simulink subsystem "ElectricalCoolingSystemSSC"  (R2022b)
settings: Solver=VariableStepAuto  StartTime=0.0  StopTime=10.0  RelTol=1e-3
undefined symbols (not defined in the file): BattTempInit, pipe, pump, radiator, T_env, T_set, tank, valve
libraries: fl_lib x101, nesl_utility_internal x25, SimscapeFluids_lib x7, slpidlib x1, simulink_extras x1
(part 2 of 3)

== system ElectricalCoolingSystemSSC/Air Stream ==
  V : Inport
  Air density [kg/m^3] : Constant  Value=1.225
  Air velocity [m/s] : Bias  Bias=5  SaturateOnIntegerOverflow=off
  Product : Product  Inputs=3
  Radiator area [m^2] : Constant  Value=radiator.area_air
  Simulink-PS Converter1 : nesl_utility_internal/Simulink-PS Converter  PhysicalDomain=network_engine_domain  SubClassName=ps_input  LeftPortType=input  RightPortType=output  PseudoPeriodic=off  Frequencies=[]  NoiseDistribution=none  NoiseParameters=[]  Unit=kg/s  AffineConversion=off  FilteringAndDerivatives=filter  SimscapeFilterOrder=1  InputFilterTimeConstant=0.01  UdotUserProvided=0
  mdot : PMIOPort  Side=Right
  wires:
  Air velocity [m/s]/1 -> Product/1
  Air density [kg/m^3]/1 -> Product/3
  Radiator area [m^2]/1 -> Product/2
  Product/1 -> Simulink-PS Converter1/1
  V/1 -> Air velocity [m/s]/1
  connections:
  mdot/RConn1 -- Simulink-PS Converter1/RConn1

== system ElectricalCoolingSystemSSC/Cold Plate ==
  One-Pass : Subsystem  VariantControl=1
  Inlet : PMIOPort  Side=Left
  Outlet : PMIOPort  Port=2  Side=Left
  Pack1 : PMIOPort  Port=3  Side=Right
  Pack2 : PMIOPort  Port=4  Side=Right
  Pack3 : PMIOPort  Port=5  Side=Right
  Pack4 : PMIOPort  Port=6  Side=Right

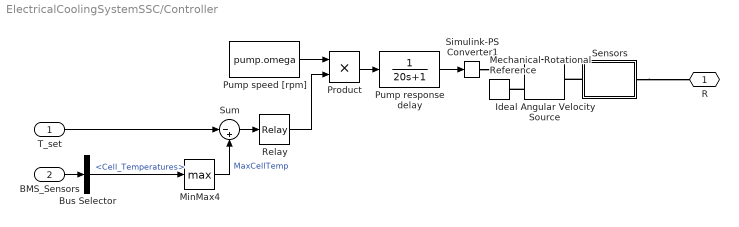
== system ElectricalCoolingSystemSSC/Controller ==
  T_set : Inport
  BMS_Sensors : Inport  Port=2
  Bus Selector : BusSelector  OutputSignals=Cell_Temperatures
  Ideal Angular Velocity Source : fl_lib/Mechanical/Mechanical Sources/Ideal Angular Velocity Source
  Mechanical Rotational Reference : fl_lib/Mechanical/Rotational Elements/Mechanical Rotational Reference
  MinMax4 : MinMax  Function=max
  Product : Product
  Pump response delay : TransferFcn  Denominator=[20 1]
  Pump speed [rpm] : Constant  Value=pump.omega
  Relay : Relay  OnSwitchValue=+1  OffSwitchValue=0.1
  Sensors : Subsystem
  Simulink-PS Converter1 : nesl_utility_internal/Simulink-PS Converter  PhysicalDomain=network_engine_domain  SubClassName=ps_input  LeftPortType=input  RightPortType=output  PseudoPeriodic=off  Frequencies=[]  NoiseDistribution=none  NoiseParameters=[]  Unit=rpm  AffineConversion=off  FilteringAndDerivatives=provide  SimscapeFilterOrder=1  InputFilterTimeConstant=0.001  UdotUserProvided=0
  Sum : Sum  Inputs=|-+
  R : PMIOPort  Side=Right
  wires:
  Pump response delay/1 -> Simulink-PS Converter1/1
  Product/1 -> Pump response delay/1
  Relay/1 -> Product/2
  Sum/1 -> Relay/1
  Pump speed [rpm]/1 -> Product/1
  T_set/1 -> Sum/1
  Bus Selector/1 -> MinMax4/1  "<Cell_Temperatures>"
  BMS_Sensors/1 -> Bus Selector/1
  MinMax4/1 -> Sum/2  "MaxCellTemp"
  connections:
  Sensors/LConn1 -- Ideal Angular Velocity Source/LConn1
  Simulink-PS Converter1/RConn1 -- Ideal Angular Velocity Source/RConn1
  Ideal Angular Velocity Source/RConn2 -- Mechanical Rotational Reference/LConn1
  Sensors/RConn1 -- R/RConn1

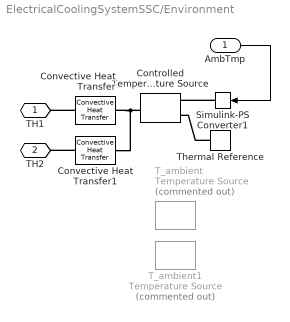
== system ElectricalCoolingSystemSSC/Environment ==
  AmbTmp : Inport
  Controlled Temperature Source : fl_lib/Thermal/Thermal Sources/Controlled Temperature Source
  Convective Heat Transfer : fl_lib/Thermal/Thermal Elements/Convective Heat Transfer  thermal_type=foundation.enum.constant_variable.constant  area=tank.area_wall/2 m^2  heat_tr_coeff=20 W/(m^2 * K)  min_heat_tr_coeff=1e-3 W/(K*m^2)  T_specify=off  T_priority=None  T=0 K  T_nominal_specify=off  T_nominal_unit=K  T_nominal_value=1  Q_specify=off  Q_priority=None  Q=0 W  Q_nominal_specify=off  Q_nominal_unit=W  Q_nominal_value=1
  Convective Heat Transfer1 : fl_lib/Thermal/Thermal Elements/Convective Heat Transfer  thermal_type=foundation.enum.constant_variable.constant  area=tank.area_wall/2 m^2  heat_tr_coeff=20 W/(m^2 * K)  min_heat_tr_coeff=1e-3 W/(K*m^2)  T_specify=off  T_priority=None  T=0 K  T_nominal_specify=off  T_nominal_unit=K  T_nominal_value=1  Q_specify=off  Q_priority=None  Q=0 W  Q_nominal_specify=off  Q_nominal_unit=W  Q_nominal_value=1
  Simulink-PS Converter1 : nesl_utility_internal/Simulink-PS Converter  PhysicalDomain=network_engine_domain  SubClassName=ps_input  LeftPortType=input  RightPortType=output  PseudoPeriodic=off  Frequencies=[]  NoiseDistribution=none  NoiseParameters=[]  Unit=1  AffineConversion=off  FilteringAndDerivatives=provide  SimscapeFilterOrder=1  InputFilterTimeConstant=0.001  UdotUserProvided=0
  T_ambient : fl_lib/Thermal/Thermal Sources/Temperature Source  Commented=on  temperature=T_env degC
  T_ambient1 : fl_lib/Thermal/Thermal Sources/Temperature Source  Commented=on  temperature=T_env degC
  Thermal Reference : fl_lib/Thermal/Thermal Elements/Thermal Reference
  TH1 : PMIOPort  Side=Left
  TH2 : PMIOPort  Port=2  Side=Left
  wires:
  AmbTmp/1 -> Simulink-PS Converter1/1
  connections:
  Convective Heat Transfer/LConn1 -- TH1/RConn1
  Convective Heat Transfer1/LConn1 -- TH2/RConn1
  Convective Heat Transfer/RConn1 -- Controlled Temperature Source/LConn1 -- Convective Heat Transfer1/RConn1
  Simulink-PS Converter1/RConn1 -- Controlled Temperature Source/RConn1
  Thermal Reference/LConn1 -- Controlled Temperature Source/RConn2

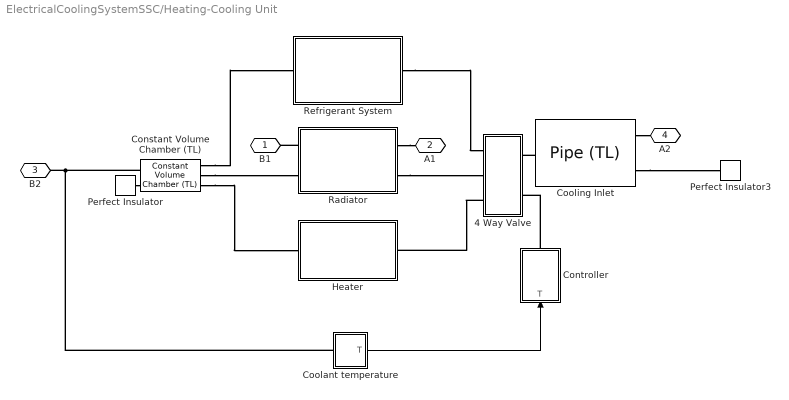
== system ElectricalCoolingSystemSSC/Heating-Cooling Unit ==
  4 Way Valve : Subsystem
  Constant Volume Chamber (TL) : fl_lib/Thermal Liquid/Elements/Constant Volume Chamber (TL)  volume=5 cm^3  num_ports=foundation.enum.num_ports.four  area_A=pipe.area m^2  area_B=pipe.area*10 m^2  area_C=pipe.area m^2  area_D=pipe.area m^2  p_I_specify=off  p_I_priority=High  p_I=0.101325 MPa  p_I_nominal_specify=off  p_I_nominal_unit=MPa  p_I_nominal_value=1  T_I_specify=on  T_I_priority=High  T_I=BattTempInit degC  T_I_nominal_specify=off  T_I_nominal_unit=K  T_I_nominal_value=1  u_chamber_specify=off  u_chamber_priority=None  u_chamber=83.90600000000001 kJ/kg  u_chamber_nominal_specify=off  u_chamber_nominal_unit=kJ/kg  u_chamber_nominal_value=1  rho_specify=off  rho_priority=None  rho=998.21 kg/m^3  rho_nominal_specify=off  rho_nominal_unit=kg/m^3  rho_nominal_value=1
      settings: InternalSimscapePortConfiguration="{\"Bottom\":[],\"Left\":[{\"id\":\"A\",\"label\":\"A\",\"type\":\"foundation.thermal_liquid.thermal_liquid\"},{\"id\":\"H\",\"label\":\"H\",\"type\":\"foundation.thermal.thermal\"}],\"Right\":[{\"id\":\"B\",\"label\":\"B\",\"type\":\"foundation.thermal_liquid.thermal_liquid\"},{\"id\":\"C\",\"label\":\"C\",\"type\":\"foundation.thermal_liquid.thermal_liquid\"},{\"id\":\"D\",\"label\":\"D\",\"type\":\"foundation.thermal_liquid.thermal_liquid\"}],\"Top\":[]}"
  Controller : Subsystem
  Coolant temperature : Subsystem
  Cooling Inlet : fl_lib/Thermal Liquid/Elements/Pipe (TL)  length=0.75 m  area=pipe.area cm^2  Dh=pipe.Dh cm  length_add=0 m  roughness=15e-6 m  Re_lam=2000  Re_tur=4000  shape_factor=64  Nu_lam=3.66  dynamic_compressibility=simscape.enum.onoff.on  inertia=simscape.enum.onoff.off  p0=0.101325 MPa  T0=BattTempInit degC  mdot0=0 kg/s
  Heater : Subsystem
  Perfect Insulator : fl_lib/Thermal/Thermal Elements/Perfect Insulator  T_specify=off  T_priority=None  T=0 K  T_nominal_specify=off  T_nominal_unit=K  T_nominal_value=1
  Perfect Insulator3 : fl_lib/Thermal/Thermal Elements/Perfect Insulator  T_specify=off  T_priority=None  T=0 K  T_nominal_specify=off  T_nominal_unit=K  T_nominal_value=1
  Radiator : Subsystem
  Refrigerant System : Subsystem
  B1 : PMIOPort  Side=Right
  A1 : PMIOPort  Port=2  Side=Left
  B2 : PMIOPort  Port=3  Side=Left
  A2 : PMIOPort  Port=4  Side=Right
  wires:
  Coolant temperature/1(T) -> Controller/1(T)
  connections:
  Constant Volume Chamber (TL)/RConn2 -- Radiator/LConn2
  4 Way Valve/LConn3 -- Heater/RConn1
  B2/RConn1 -- Coolant temperature/LConn1 -- Constant Volume Chamber (TL)/LConn1
  Constant Volume Chamber (TL)/RConn3 -- Heater/LConn1
  Radiator/LConn1 -- B1/RConn1
  Refrigerant System/RConn1 -- 4 Way Valve/LConn1
  Radiator/RConn1 -- A1/RConn1
  Cooling Inlet/LConn1 -- A2/RConn1
  Cooling Inlet/RConn1 -- 4 Way Valve/RConn1
  Radiator/RConn2 -- 4 Way Valve/LConn2
  Controller/RConn1 -- 4 Way Valve/RConn2
  Constant Volume Chamber (TL)/RConn1 -- Refrigerant System/LConn1
  Cooling Inlet/LConn2 -- Perfect Insulator3/LConn1
  Perfect Insulator/LConn1 -- Constant Volume Chamber (TL)/LConn2

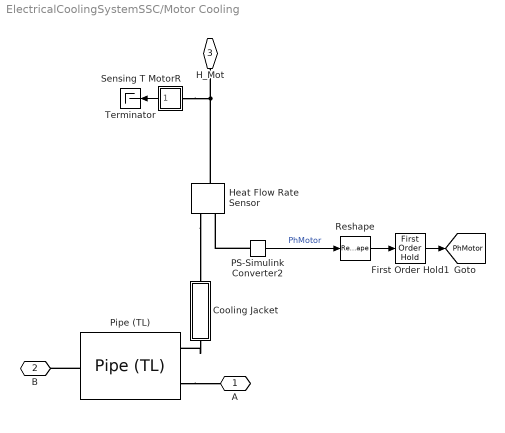
== system ElectricalCoolingSystemSSC/Motor Cooling ==
  Cooling Jacket : Subsystem
  First Order Hold1 : FirstOrderHold  ErrorTolerance=inf  AllowContinuousInput=on
  Heat Flow Rate Sensor : fl_lib/Thermal/Thermal Sensors/Heat Flow Rate Sensor
  PS-Simulink Converter2 : nesl_utility_internal/PS-Simulink Converter  PhysicalDomain=network_engine_domain  SubClassName=ps_output  LeftPortType=input  RightPortType=output  PseudoPeriodic=off  Frequencies=[]  VectorFormat=inherit  Unit=inherit  AffineConversion=off
  Pipe (TL) : fl_lib/Thermal Liquid/Elements/Pipe (TL)  length=pipe.length cm  area=pipe.area cm^2  Dh=pipe.Dh cm  length_add=0 m  roughness=15e-6 m  Re_lam=2000  Re_tur=4000  shape_factor=64  Nu_lam=3.66  dynamic_compressibility=simscape.enum.onoff.on  inertia=simscape.enum.onoff.off  p0=0.101325 MPa  T0=BattTempInit degC  mdot0=0 kg/s
  Reshape : Reshape
  Sensing T MotorR : Subsystem
  Terminator : Terminator
  A : PMIOPort  Side=Left
  B : PMIOPort  Port=2  Side=Right
  H_Mot : PMIOPort  Port=3  Side=Right
  tag scope: PhMotor=global
  wires:
  Sensing T MotorR/1(T) -> Terminator/1
  PS-Simulink Converter2/1 -> Reshape/1  "PhMotor"
  Reshape/1 -> First Order Hold1/1
  First Order Hold1/1 -> [PhMotor]
  connections:
  Pipe (TL)/RConn1 -- B/RConn1
  Pipe (TL)/LConn1 -- A/RConn1
  Sensing T MotorR/LConn1 -- H_Mot/RConn1 -- Heat Flow Rate Sensor/LConn1
  Cooling Jacket/LConn1 -- Pipe (TL)/LConn2
  PS-Simulink Converter2/LConn1 -- Heat Flow Rate Sensor/RConn1
  Heat Flow Rate Sensor/RConn2 -- Cooling Jacket/RConn1

== system ElectricalCoolingSystemSSC/Power Sensor ==
  First Order Hold1 : FirstOrderHold  ErrorTolerance=inf  AllowContinuousInput=on
  Heat Flow Rate Sensor : fl_lib/Thermal/Thermal Sensors/Heat Flow Rate Sensor
  PS-Simulink Converter2 : nesl_utility_internal/PS-Simulink Converter  PhysicalDomain=network_engine_domain  SubClassName=ps_output  LeftPortType=input  RightPortType=output  PseudoPeriodic=off  Frequencies=[]  VectorFormat=inherit  Unit=inherit  AffineConversion=off
  Reshape : Reshape
  A : PMIOPort  Side=Left
  B : PMIOPort  Port=2  Side=Right
  tag scope: Ph1=global
  wires:
  PS-Simulink Converter2/1 -> Reshape/1  "Ph1"
  Reshape/1 -> First Order Hold1/1
  First Order Hold1/1 -> [Ph1]
  connections:
  PS-Simulink Converter2/LConn1 -- Heat Flow Rate Sensor/RConn1
  Heat Flow Rate Sensor/LConn1 -- A/RConn1
  Heat Flow Rate Sensor/RConn2 -- B/RConn1

== system ElectricalCoolingSystemSSC/Power Sensor1 ==
  First Order Hold1 : FirstOrderHold  ErrorTolerance=inf  AllowContinuousInput=on
  Mass & Energy Flow Rate Sensor (TL) : fl_lib/Thermal Liquid/Sensors/Mass & Energy Flow Rate Sensor (TL)
      settings: InternalSimscapePortConfiguration="{\"Bottom\":[],\"Left\":[{\"id\":\"A\",\"label\":\"A\",\"type\":\"foundation.thermal_liquid.thermal_liquid\"}],\"Right\":[{\"id\":\"B\",\"label\":\"B\",\"type\":\"foundation.thermal_liquid.thermal_liquid\"},{\"id\":\"M\",\"label\":\"M\",\"type\":\"output\"},{\"id\":\"PHI\",\"label\":\"Phi\",\"type\":\"output\"}],\"Top\":[]}"
  PS-Simulink Converter2 : nesl_utility_internal/PS-Simulink Converter  PhysicalDomain=network_engine_domain  SubClassName=ps_output  LeftPortType=input  RightPortType=output  PseudoPeriodic=off  Frequencies=[]  VectorFormat=inherit  Unit=inherit  AffineConversion=off
  Reshape : Reshape
  B : PMIOPort  Side=Left
  A : PMIOPort  Port=2  Side=Right
  tag scope: PcpOutlet=global
  wires:
  PS-Simulink Converter2/1 -> Reshape/1  "PcpOutlet"
  Reshape/1 -> First Order Hold1/1
  First Order Hold1/1 -> [PcpOutlet]
  connections:
  Mass & Energy Flow Rate Sensor (TL)/RConn1 -- B/RConn1
  Mass & Energy Flow Rate Sensor (TL)/RConn3 -- PS-Simulink Converter2/LConn1
  Mass & Energy Flow Rate Sensor (TL)/LConn1 -- A/RConn1

== system ElectricalCoolingSystemSSC/Power Sensor2 ==
  First Order Hold1 : FirstOrderHold  ErrorTolerance=inf  AllowContinuousInput=on
  Mass & Energy Flow Rate Sensor (TL) : fl_lib/Thermal Liquid/Sensors/Mass & Energy Flow Rate Sensor (TL)
      settings: InternalSimscapePortConfiguration="{\"Bottom\":[],\"Left\":[{\"id\":\"A\",\"label\":\"A\",\"type\":\"foundation.thermal_liquid.thermal_liquid\"}],\"Right\":[{\"id\":\"B\",\"label\":\"B\",\"type\":\"foundation.thermal_liquid.thermal_liquid\"},{\"id\":\"M\",\"label\":\"M\",\"type\":\"output\"},{\"id\":\"PHI\",\"label\":\"Phi\",\"type\":\"output\"}],\"Top\":[]}"
  PS-Simulink Converter2 : nesl_utility_internal/PS-Simulink Converter  PhysicalDomain=network_engine_domain  SubClassName=ps_output  LeftPortType=input  RightPortType=output  PseudoPeriodic=off  Frequencies=[]  VectorFormat=inherit  Unit=inherit  AffineConversion=off
  Reshape : Reshape
  B : PMIOPort  Side=Left
  A : PMIOPort  Port=2  Side=Right
  tag scope: PhcuOut=global
  wires:
  PS-Simulink Converter2/1 -> Reshape/1  "PhcuOut"
  Reshape/1 -> First Order Hold1/1
  First Order Hold1/1 -> [PhcuOut]
  connections:
  Mass & Energy Flow Rate Sensor (TL)/LConn1 -- A/RConn1
  Mass & Energy Flow Rate Sensor (TL)/RConn3 -- PS-Simulink Converter2/LConn1
  Mass & Energy Flow Rate Sensor (TL)/RConn1 -- B/RConn1

== system ElectricalCoolingSystemSSC/Power Sensor3 ==
  First Order Hold1 : FirstOrderHold  ErrorTolerance=inf  AllowContinuousInput=on
  Mass & Energy Flow Rate Sensor (TL) : fl_lib/Thermal Liquid/Sensors/Mass & Energy Flow Rate Sensor (TL)
      settings: InternalSimscapePortConfiguration="{\"Bottom\":[],\"Left\":[{\"id\":\"A\",\"label\":\"A\",\"type\":\"foundation.thermal_liquid.thermal_liquid\"}],\"Right\":[{\"id\":\"B\",\"label\":\"B\",\"type\":\"foundation.thermal_liquid.thermal_liquid\"},{\"id\":\"M\",\"label\":\"M\",\"type\":\"output\"},{\"id\":\"PHI\",\"label\":\"Phi\",\"type\":\"output\"}],\"Top\":[]}"
  PS-Simulink Converter2 : nesl_utility_internal/PS-Simulink Converter  PhysicalDomain=network_engine_domain  SubClassName=ps_output  LeftPortType=input  RightPortType=output  PseudoPeriodic=off  Frequencies=[]  VectorFormat=inherit  Unit=inherit  AffineConversion=off
  Reshape : Reshape
  B : PMIOPort  Side=Left
  A : PMIOPort  Port=2  Side=Right
  tag scope: PhcuIn=global
  wires:
  PS-Simulink Converter2/1 -> Reshape/1  "PhcuIn"
  Reshape/1 -> First Order Hold1/1
  First Order Hold1/1 -> [PhcuIn]
  connections:
  Mass & Energy Flow Rate Sensor (TL)/LConn1 -- A/RConn1
  Mass & Energy Flow Rate Sensor (TL)/RConn3 -- PS-Simulink Converter2/LConn1
  Mass & Energy Flow Rate Sensor (TL)/RConn1 -- B/RConn1

== system ElectricalCoolingSystemSSC/Power Sensor4 ==
  First Order Hold1 : FirstOrderHold  ErrorTolerance=inf  AllowContinuousInput=on
  Mass & Energy Flow Rate Sensor (TL) : fl_lib/Thermal Liquid/Sensors/Mass & Energy Flow Rate Sensor (TL)
      settings: InternalSimscapePortConfiguration="{\"Bottom\":[],\"Left\":[{\"id\":\"A\",\"label\":\"A\",\"type\":\"foundation.thermal_liquid.thermal_liquid\"}],\"Right\":[{\"id\":\"B\",\"label\":\"B\",\"type\":\"foundation.thermal_liquid.thermal_liquid\"},{\"id\":\"M\",\"label\":\"M\",\"type\":\"output\"},{\"id\":\"PHI\",\"label\":\"Phi\",\"type\":\"output\"}],\"Top\":[]}"
  PS-Simulink Converter2 : nesl_utility_internal/PS-Simulink Converter  PhysicalDomain=network_engine_domain  SubClassName=ps_output  LeftPortType=input  RightPortType=output  PseudoPeriodic=off  Frequencies=[]  VectorFormat=inherit  Unit=inherit  AffineConversion=off
  Reshape : Reshape
  B : PMIOPort  Side=Left
  A : PMIOPort  Port=2  Side=Right
  tag scope: PMotOut=global
  wires:
  PS-Simulink Converter2/1 -> Reshape/1  "PMotOut"
  Reshape/1 -> First Order Hold1/1
  First Order Hold1/1 -> [PMotOut]
  connections:
  Mass & Energy Flow Rate Sensor (TL)/LConn1 -- A/RConn1
  Mass & Energy Flow Rate Sensor (TL)/RConn3 -- PS-Simulink Converter2/LConn1
  Mass & Energy Flow Rate Sensor (TL)/RConn1 -- B/RConn1

== system ElectricalCoolingSystemSSC/Power Sensor6 ==
  First Order Hold1 : FirstOrderHold  ErrorTolerance=inf  AllowContinuousInput=on
  Heat Flow Rate Sensor : fl_lib/Thermal/Thermal Sensors/Heat Flow Rate Sensor
  PS-Simulink Converter2 : nesl_utility_internal/PS-Simulink Converter  PhysicalDomain=network_engine_domain  SubClassName=ps_output  LeftPortType=input  RightPortType=output  PseudoPeriodic=off  Frequencies=[]  VectorFormat=inherit  Unit=inherit  AffineConversion=off
  Reshape : Reshape
  A : PMIOPort  Side=Left
  B : PMIOPort  Port=2  Side=Right
  tag scope: Ph2=global
  wires:
  PS-Simulink Converter2/1 -> Reshape/1
  Reshape/1 -> First Order Hold1/1
  First Order Hold1/1 -> [Ph2]
  connections:
  Heat Flow Rate Sensor/RConn2 -- B/RConn1
  Heat Flow Rate Sensor/LConn1 -- A/RConn1
  PS-Simulink Converter2/LConn1 -- Heat Flow Rate Sensor/RConn1

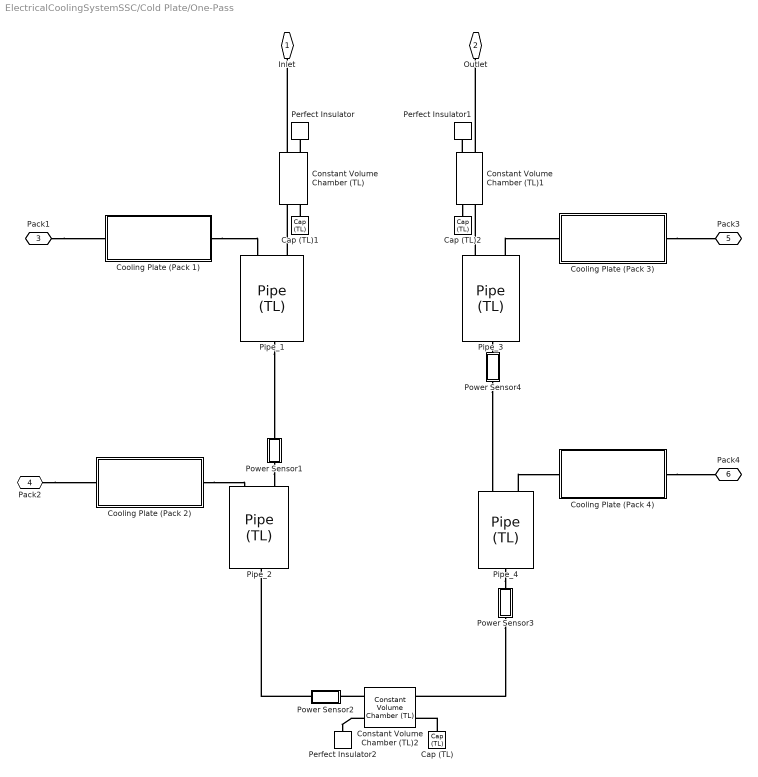
== system ElectricalCoolingSystemSSC/Cold Plate/One-Pass ==
  Cap (TL) : fl_lib/Thermal Liquid/Elements/Cap (TL)  p_specify=off  p_priority=None  p=0.101325 MPa  p_nominal_specify=off  p_nominal_unit=MPa  p_nominal_value=1  T_specify=off  T_priority=None  T=293.15 K  T_nominal_specify=off  T_nominal_unit=K  T_nominal_value=1
      settings: InternalSimscapePortConfiguration="{\"Bottom\":[],\"Left\":[{\"id\":\"A\",\"label\":\"\",\"type\":\"foundation.thermal_liquid.thermal_liquid\"}],\"Right\":[],\"Top\":[]}"
  Cap (TL)1 : fl_lib/Thermal Liquid/Elements/Cap (TL)  p_specify=off  p_priority=None  p=0.101325 MPa  p_nominal_specify=off  p_nominal_unit=MPa  p_nominal_value=1  T_specify=off  T_priority=None  T=293.15 K  T_nominal_specify=off  T_nominal_unit=K  T_nominal_value=1
      settings: InternalSimscapePortConfiguration="{\"Bottom\":[],\"Left\":[{\"id\":\"A\",\"label\":\"\",\"type\":\"foundation.thermal_liquid.thermal_liquid\"}],\"Right\":[],\"Top\":[]}"
  Cap (TL)2 : fl_lib/Thermal Liquid/Elements/Cap (TL)  p_specify=off  p_priority=None  p=0.101325 MPa  p_nominal_specify=off  p_nominal_unit=MPa  p_nominal_value=1  T_specify=off  T_priority=None  T=293.15 K  T_nominal_specify=off  T_nominal_unit=K  T_nominal_value=1
      settings: InternalSimscapePortConfiguration="{\"Bottom\":[],\"Left\":[{\"id\":\"A\",\"label\":\"\",\"type\":\"foundation.thermal_liquid.thermal_liquid\"}],\"Right\":[],\"Top\":[]}"
  Constant Volume Chamber (TL) : fl_lib/Thermal Liquid/Elements/Constant Volume Chamber (TL)  volume=0.001 m^3  num_ports=foundation.enum.num_ports.three  area_A=3 cm^2  area_B=3 cm^2  area_C=3 cm^2  area_D=0.01 m^2  p_I_specify=off  p_I_priority=High  p_I=0.101325 MPa  p_I_nominal_specify=off  p_I_nominal_unit=MPa  p_I_nominal_value=1  T_I_specify=on  T_I_priority=High  T_I=BattTempInit degC  T_I_nominal_specify=off  T_I_nominal_unit=K  T_I_nominal_value=1  u_chamber_specify=off  u_chamber_priority=None  u_chamber=83.90600000000001 kJ/kg  u_chamber_nominal_specify=off  u_chamber_nominal_unit=kJ/kg  u_chamber_nominal_value=1  rho_specify=off  rho_priority=None  rho=998.21 kg/m^3  rho_nominal_specify=off  rho_nominal_unit=kg/m^3  rho_nominal_value=1
      settings: InternalSimscapePortConfiguration="{\"Bottom\":[],\"Left\":[{\"id\":\"A\",\"label\":\"A\",\"type\":\"foundation.thermal_liquid.thermal_liquid\"},{\"id\":\"H\",\"label\":\"H\",\"type\":\"foundation.thermal.thermal\"}],\"Right\":[{\"id\":\"B\",\"label\":\"B\",\"type\":\"foundation.thermal_liquid.thermal_liquid\"},{\"id\":\"C\",\"label\":\"C\",\"type\":\"foundation.thermal_liquid.thermal_liquid\"}],\"Top\":[]}"
  Constant Volume Chamber (TL)1 : fl_lib/Thermal Liquid/Elements/Constant Volume Chamber (TL)  volume=0.001 m^3  num_ports=foundation.enum.num_ports.three  area_A=3 cm^2  area_B=3 cm^2  area_C=3 cm^2  area_D=0.01 m^2  p_I_specify=off  p_I_priority=High  p_I=0.101325 MPa  p_I_nominal_specify=off  p_I_nominal_unit=MPa  p_I_nominal_value=1  T_I_specify=on  T_I_priority=High  T_I=BattTempInit degC  T_I_nominal_specify=off  T_I_nominal_unit=K  T_I_nominal_value=1  u_chamber_specify=off  u_chamber_priority=None  u_chamber=83.90600000000001 kJ/kg  u_chamber_nominal_specify=off  u_chamber_nominal_unit=kJ/kg  u_chamber_nominal_value=1  rho_specify=off  rho_priority=None  rho=998.21 kg/m^3  rho_nominal_specify=off  rho_nominal_unit=kg/m^3  rho_nominal_value=1
      settings: InternalSimscapePortConfiguration="{\"Bottom\":[],\"Left\":[{\"id\":\"A\",\"label\":\"A\",\"type\":\"foundation.thermal_liquid.thermal_liquid\"},{\"id\":\"H\",\"label\":\"H\",\"type\":\"foundation.thermal.thermal\"}],\"Right\":[{\"id\":\"B\",\"label\":\"B\",\"type\":\"foundation.thermal_liquid.thermal_liquid\"},{\"id\":\"C\",\"label\":\"C\",\"type\":\"foundation.thermal_liquid.thermal_liquid\"}],\"Top\":[]}"
  Constant Volume Chamber (TL)2 : fl_lib/Thermal Liquid/Elements/Constant Volume Chamber (TL)  volume=0.001 m^3  num_ports=foundation.enum.num_ports.three  area_A=3 cm^2  area_B=3 cm^2  area_C=3 cm^2  area_D=0.01 m^2  p_I_specify=off  p_I_priority=High  p_I=0.101325 MPa  p_I_nominal_specify=off  p_I_nominal_unit=MPa  p_I_nominal_value=1  T_I_specify=on  T_I_priority=High  T_I=BattTempInit degC  T_I_nominal_specify=off  T_I_nominal_unit=K  T_I_nominal_value=1  u_chamber_specify=off  u_chamber_priority=None  u_chamber=83.90600000000001 kJ/kg  u_chamber_nominal_specify=off  u_chamber_nominal_unit=kJ/kg  u_chamber_nominal_value=1  rho_specify=off  rho_priority=None  rho=998.21 kg/m^3  rho_nominal_specify=off  rho_nominal_unit=kg/m^3  rho_nominal_value=1
      settings: InternalSimscapePortConfiguration="{\"Bottom\":[],\"Left\":[{\"id\":\"A\",\"label\":\"A\",\"type\":\"foundation.thermal_liquid.thermal_liquid\"},{\"id\":\"H\",\"label\":\"H\",\"type\":\"foundation.thermal.thermal\"}],\"Right\":[{\"id\":\"B\",\"label\":\"B\",\"type\":\"foundation.thermal_liquid.thermal_liquid\"},{\"id\":\"C\",\"label\":\"C\",\"type\":\"foundation.thermal_liquid.thermal_liquid\"}],\"Top\":[]}"
  Cooling Plate (Pack 1) : Subsystem
  Cooling Plate (Pack 2) : Subsystem
  Cooling Plate (Pack 3) : Subsystem
  Cooling Plate (Pack 4) : Subsystem
  Perfect Insulator : fl_lib/Thermal/Thermal Elements/Perfect Insulator  T_specify=off  T_priority=None  T=0 K  T_nominal_specify=off  T_nominal_unit=K  T_nominal_value=1
  Perfect Insulator1 : fl_lib/Thermal/Thermal Elements/Perfect Insulator  T_specify=off  T_priority=None  T=0 K  T_nominal_specify=off  T_nominal_unit=K  T_nominal_value=1
  Perfect Insulator2 : fl_lib/Thermal/Thermal Elements/Perfect Insulator  T_specify=off  T_priority=None  T=0 K  T_nominal_specify=off  T_nominal_unit=K  T_nominal_value=1
  Pipe_{1..4} (4 alike) : fl_lib/Thermal Liquid/Elements/Pipe (TL)  length=1.5 m  area=3*2 cm^2  Dh=0.92*sqrt(2) cm  length_add=0 m  roughness=15e-6 m  Re_lam=2000  Re_tur=4000  shape_factor=64  Nu_lam=3.66  dynamic_compressibility=simscape.enum.onoff.on  inertia=simscape.enum.onoff.off  p0=0.101325 MPa  T0=BattTempInit degC  mdot0=0 kg/s
  Power Sensor1 : Subsystem
  Power Sensor2 : Subsystem
  Power Sensor3 : Subsystem
  Power Sensor4 : Subsystem
  Inlet : PMIOPort  Side=Left
  Outlet : PMIOPort  Port=2  Side=Left
  Pack1 : PMIOPort  Port=3  Side=Right
  Pack2 : PMIOPort  Port=4  Side=Right
  Pack3 : PMIOPort  Port=5  Side=Right
  Pack4 : PMIOPort  Port=6  Side=Right
  connections:
  Constant Volume Chamber (TL)1/RConn2 -- Cap (TL)2/LConn1
  Cap (TL)1/LConn1 -- Constant Volume Chamber (TL)/RConn2
  Cap (TL)/LConn1 -- Constant Volume Chamber (TL)2/RConn2
  Pipe_3/RConn1 -- Power Sensor4/RConn1
  Constant Volume Chamber (TL)2/LConn1 -- Power Sensor2/RConn1
  Constant Volume Chamber (TL)/LConn1 -- Inlet/RConn1
  Constant Volume Chamber (TL)1/LConn2 -- Perfect Insulator1/LConn1
  Power Sensor3/LConn1 -- Constant Volume Chamber (TL)2/RConn1
  Constant Volume Chamber (TL)1/LConn1 -- Outlet/RConn1
  Pack1/RConn1 -- Cooling Plate (Pack 1)/RConn1
  Pack2/RConn1 -- Cooling Plate (Pack 2)/RConn1
  Pipe_1/RConn1 -- Power Sensor1/RConn1
  Pipe_3/LConn1 -- Constant Volume Chamber (TL)1/RConn1
  Pipe_3/LConn2 -- Cooling Plate (Pack 3)/LConn1
  Pipe_4/LConn2 -- Cooling Plate (Pack 4)/LConn1
  Cooling Plate (Pack 1)/LConn1 -- Pipe_1/LConn2
  Cooling Plate (Pack 2)/LConn1 -- Pipe_2/LConn2
  Cooling Plate (Pack 3)/RConn1 -- Pack3/RConn1
  Cooling Plate (Pack 4)/RConn1 -- Pack4/RConn1
  Power Sensor1/LConn1 -- Pipe_2/LConn1
  Power Sensor4/LConn1 -- Pipe_4/LConn1
  Power Sensor2/LConn1 -- Pipe_2/RConn1
  Pipe_4/RConn1 -- Power Sensor3/RConn1
  Constant Volume Chamber (TL)2/LConn2 -- Perfect Insulator2/LConn1
  Pipe_1/LConn1 -- Constant Volume Chamber (TL)/RConn1
  Constant Volume Chamber (TL)/LConn2 -- Perfect Insulator/LConn1

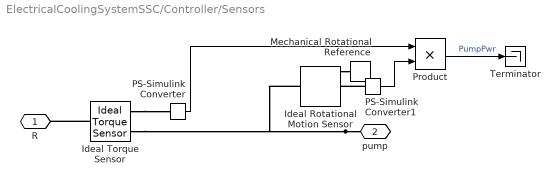
== system ElectricalCoolingSystemSSC/Controller/Sensors ==
  Ideal Rotational Motion Sensor : fl_lib/Mechanical/Mechanical Sensors/Ideal Rotational Motion Sensor  reference=foundation.enum.MeasurementReference.difference  acceleration_port=false  velocity_port=true  position_port=true  wrap_angle=simscape.enum.onoff.off  offset=0 rad
  Ideal Torque Sensor : fl_lib/Mechanical/Mechanical Sensors/Ideal Torque Sensor
  Mechanical Rotational Reference : fl_lib/Mechanical/Rotational Elements/Mechanical Rotational Reference
  PS-Simulink Converter : nesl_utility_internal/PS-Simulink Converter  PhysicalDomain=network_engine_domain  SubClassName=ps_output  LeftPortType=input  RightPortType=output  PseudoPeriodic=off  Frequencies=[]  VectorFormat=1-D array  Unit=N*m  AffineConversion=off
  PS-Simulink Converter1 : nesl_utility_internal/PS-Simulink Converter  PhysicalDomain=network_engine_domain  SubClassName=ps_output  LeftPortType=input  RightPortType=output  PseudoPeriodic=off  Frequencies=[]  VectorFormat=1-D array  Unit=rad/s  AffineConversion=off
  Product : Product
  Terminator : Terminator
  R : PMIOPort  Side=Left
  pump : PMIOPort  Port=2  Side=Right
  wires:
  PS-Simulink Converter/1 -> Product/1
  PS-Simulink Converter1/1 -> Product/2
  Product/1 -> Terminator/1  "PumpPwr"
  connections:
  Ideal Rotational Motion Sensor/RConn1 -- Mechanical Rotational Reference/LConn1
  Ideal Torque Sensor/LConn1 -- R/RConn1
  Ideal Torque Sensor/RConn2 -- PS-Simulink Converter/LConn1
  PS-Simulink Converter1/LConn1 -- Ideal Rotational Motion Sensor/RConn2
  pump/RConn1 -- Ideal Rotational Motion Sensor/LConn1 -- Ideal Torque Sensor/RConn1

== system ElectricalCoolingSystemSSC/Heating-Cooling Unit/4 Way Valve ==
  Variable Area Orifice (TL) : SimscapeFluids_lib/Thermal Liquid/Valves & Orifices/Orifice (TL)  orifice_type=foundation.enum.constant_variable.variable  constant_orifice_spec=fluids.thermal_liquid.valves.enum.ConstantOrificeSpec.Area  variable_orifice_spec=2  orifice_area_constant=1e-3 m^2  p_diff_TLU_constant=[-4, -3, -2, -1, -.5, 0, .5, 1, 2, 3, 4] MPa  vol_flow_TLU_constant=[-2.44, -2.12, -1.68, -1.22, -.84, 0, .85, 1.21, 1.7, 2.09, 2.41] .* 1e-3 m^3/s  mdot_TLU_constant=[-2.44, -2.12, -1.68, -1.22, -.84, 0, .85, 1.21, 1.7, 2.09, 2.41] kg/s  S_min=5e-06 mm  del_S=0.004999995 m  open_orientation=1  area_max=1e-4 m^2  area_leak=1e-10 m^2  S_TLU=[2 3] mm  orifice_area_TLU=[valve.opening, valve.area_leak] cm^2  Cd=0.7  Re_c=12  smoothing_factor=0.01  pressure_recovery=1  S_flow_TLU=[-2 0 2 5 15] mm  p_diff_TLU=[-.1, .3, .5, .7] MPa  vol_flow_TLU=1e-3 * [1.7e-05, 2e-05, 2.6e-05; .0035, .0045, .0053; .7, .9, 1.06; 1.96, 2.5, 3; 6, 7.7, 9.13] m^3/s  mdot_TLU=[-1e-05, 1.7e-05, 2e-05, 2.6e-05; -.002, .0035, .0045, .0053; -.4, .7, .9, 1.06; -1.13, 1.96, 2.5, 3; -3.45, 6, 7.7, 9.13] kg/s  T_ref_in=293.15 K  p_ref_in=0.101325 MPa  area=valve.area cm^2  mdot_A_specify=off  mdot_A_priority=None  mdot_A=1 kg/s  mdot_A_nominal_specify=off  mdot_A_nominal_unit=kg/s  mdot_A_nominal_value=1  mdot_B_specify=off  mdot_B_priority=None  mdot_B=0 kg/s  mdot_B_nominal_specify=off  mdot_B_nominal_unit=kg/s  mdot_B_nominal_value=1  Phi_A_specify=off  Phi_A_priority=None  Phi_A=0 kW  Phi_A_nominal_specify=off  Phi_A_nominal_unit=kW  Phi_A_nominal_value=1  Phi_B_specify=off  Phi_B_priority=None  Phi_B=0 kW  Phi_B_nominal_specify=off  Phi_B_nominal_unit=kW  Phi_B_nominal_value=1
      settings: InternalSimscapePortConfiguration="{\"Bottom\":[],\"Left\":[{\"id\":\"A\",\"label\":\"A\",\"type\":\"foundation.thermal_liquid.thermal_liquid\"},{\"id\":\"S\",\"label\":\"S\",\"type\":\"input\"}],\"Right\":[{\"id\":\"B\",\"label\":\"B\",\"type\":\"foundation.thermal_liquid.thermal_liquid\"}],\"Top\":[]}"
  Variable Area Orifice (TL)1 : SimscapeFluids_lib/Thermal Liquid/Valves & Orifices/Orifice (TL)  orifice_type=foundation.enum.constant_variable.variable  constant_orifice_spec=fluids.thermal_liquid.valves.enum.ConstantOrificeSpec.Area  variable_orifice_spec=fluids.thermal_liquid.valves.enum.orifice_spec.table1D_area_opening  orifice_area_constant=1e-3 m^2  p_diff_TLU_constant=[-4, -3, -2, -1, -.5, 0, .5, 1, 2, 3, 4] MPa  vol_flow_TLU_constant=[-2.44, -2.12, -1.68, -1.22, -.84, 0, .85, 1.21, 1.7, 2.09, 2.41] .* 1e-3 m^3/s  mdot_TLU_constant=[-2.44, -2.12, -1.68, -1.22, -.84, 0, .85, 1.21, 1.7, 2.09, 2.41] kg/s  S_min=5e-06 mm  del_S=0.004999995 m  open_orientation=simscape.enum.posneg.positive  area_max=1e-4 m^2  area_leak=1e-10 m^2  S_TLU=[2 3 6 7] mm  orifice_area_TLU=[valve.area_leak, valve.opening, valve.opening, valve.area_leak] cm^2  Cd=0.7  Re_c=12  smoothing_factor=0.01  pressure_recovery=simscape.enum.onoff.on  S_flow_TLU=[-2 0 2 5 15] mm  p_diff_TLU=[-.1, .3, .5, .7] MPa  vol_flow_TLU=1e-3 * [1.7e-05, 2e-05, 2.6e-05; .0035, .0045, .0053; .7, .9, 1.06; 1.96, 2.5, 3; 6, 7.7, 9.13] m^3/s  mdot_TLU=[-1e-05, 1.7e-05, 2e-05, 2.6e-05; -.002, .0035, .0045, .0053; -.4, .7, .9, 1.06; -1.13, 1.96, 2.5, 3; -3.45, 6, 7.7, 9.13] kg/s  T_ref_in=293.15 K  p_ref_in=0.101325 MPa  area=valve.area cm^2  mdot_A_specify=off  mdot_A_priority=None  mdot_A=1 kg/s  mdot_A_nominal_specify=off  mdot_A_nominal_unit=kg/s  mdot_A_nominal_value=1  mdot_B_specify=off  mdot_B_priority=None  mdot_B=0 kg/s  mdot_B_nominal_specify=off  mdot_B_nominal_unit=kg/s  mdot_B_nominal_value=1  Phi_A_specify=off  Phi_A_priority=None  Phi_A=0 kW  Phi_A_nominal_specify=off  Phi_A_nominal_unit=kW  Phi_A_nominal_value=1  Phi_B_specify=off  Phi_B_priority=None  Phi_B=0 kW  Phi_B_nominal_specify=off  Phi_B_nominal_unit=kW  Phi_B_nominal_value=1
      settings: InternalSimscapePortConfiguration="{\"Bottom\":[],\"Left\":[{\"id\":\"A\",\"label\":\"A\",\"type\":\"foundation.thermal_liquid.thermal_liquid\"},{\"id\":\"S\",\"label\":\"S\",\"type\":\"input\"}],\"Right\":[{\"id\":\"B\",\"label\":\"B\",\"type\":\"foundation.thermal_liquid.thermal_liquid\"}],\"Top\":[]}"
  Variable Area Orifice (TL)2 : SimscapeFluids_lib/Thermal Liquid/Valves & Orifices/Orifice (TL)  orifice_type=foundation.enum.constant_variable.variable  constant_orifice_spec=fluids.thermal_liquid.valves.enum.ConstantOrificeSpec.Area  variable_orifice_spec=fluids.thermal_liquid.valves.enum.orifice_spec.table1D_area_opening  orifice_area_constant=1e-3 m^2  p_diff_TLU_constant=[-4, -3, -2, -1, -.5, 0, .5, 1, 2, 3, 4] MPa  vol_flow_TLU_constant=[-2.44, -2.12, -1.68, -1.22, -.84, 0, .85, 1.21, 1.7, 2.09, 2.41] .* 1e-3 m^3/s  mdot_TLU_constant=[-2.44, -2.12, -1.68, -1.22, -.84, 0, .85, 1.21, 1.7, 2.09, 2.41] kg/s  S_min=5e-06 mm  del_S=0.004999995 m  open_orientation=simscape.enum.posneg.positive  area_max=1e-4 m^2  area_leak=1e-10 m^2  S_TLU=[6 7] mm  orifice_area_TLU=[valve.area_leak, valve.opening] cm^2  Cd=0.7  Re_c=12  smoothing_factor=0.01  pressure_recovery=simscape.enum.onoff.on  S_flow_TLU=[-2 0 2 5 15] mm  p_diff_TLU=[-.1, .3, .5, .7] MPa  vol_flow_TLU=1e-3 * [1.7e-05, 2e-05, 2.6e-05; .0035, .0045, .0053; .7, .9, 1.06; 1.96, 2.5, 3; 6, 7.7, 9.13] m^3/s  mdot_TLU=[-1e-05, 1.7e-05, 2e-05, 2.6e-05; -.002, .0035, .0045, .0053; -.4, .7, .9, 1.06; -1.13, 1.96, 2.5, 3; -3.45, 6, 7.7, 9.13] kg/s  T_ref_in=293.15 K  p_ref_in=0.101325 MPa  area=valve.area cm^2  mdot_A_specify=off  mdot_A_priority=None  mdot_A=1 kg/s  mdot_A_nominal_specify=off  mdot_A_nominal_unit=kg/s  mdot_A_nominal_value=1  mdot_B_specify=off  mdot_B_priority=None  mdot_B=0 kg/s  mdot_B_nominal_specify=off  mdot_B_nominal_unit=kg/s  mdot_B_nominal_value=1  Phi_A_specify=off  Phi_A_priority=None  Phi_A=0 kW  Phi_A_nominal_specify=off  Phi_A_nominal_unit=kW  Phi_A_nominal_value=1  Phi_B_specify=off  Phi_B_priority=None  Phi_B=0 kW  Phi_B_nominal_specify=off  Phi_B_nominal_unit=kW  Phi_B_nominal_value=1
      settings: InternalSimscapePortConfiguration="{\"Bottom\":[],\"Left\":[{\"id\":\"A\",\"label\":\"A\",\"type\":\"foundation.thermal_liquid.thermal_liquid\"},{\"id\":\"S\",\"label\":\"S\",\"type\":\"input\"}],\"Right\":[{\"id\":\"B\",\"label\":\"B\",\"type\":\"foundation.thermal_liquid.thermal_liquid\"}],\"Top\":[]}"
  T1 : PMIOPort  Side=Left
  A : PMIOPort  Port=2  Side=Right
  T2 : PMIOPort  Port=3  Side=Left
  T3 : PMIOPort  Port=4  Side=Left
  S : PMIOPort  Port=5  Side=Right
  connections:
  Variable Area Orifice (TL)1/LConn2 -- Variable Area Orifice (TL)2/LConn2 -- S/RConn1 -- Variable Area Orifice (TL)/LConn2
  Variable Area Orifice (TL)2/LConn1 -- A/RConn1 -- Variable Area Orifice (TL)1/LConn1 -- Variable Area Orifice (TL)/LConn1
  Variable Area Orifice (TL)/RConn1 -- T1/RConn1
  Variable Area Orifice (TL)2/RConn1 -- T3/RConn1
  Variable Area Orifice (TL)1/RConn1 -- T2/RConn1

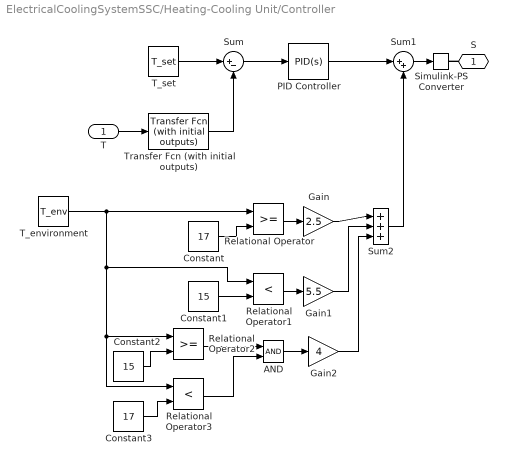
== system ElectricalCoolingSystemSSC/Heating-Cooling Unit/Controller ==
  T : Inport
  AND : Logic  IconShape=distinctive  AllPortsSameDT=off  OutDataTypeStr=boolean
  Constant : Constant  Value=17
  Constant1 : Constant  Value=15
  Constant2 : Constant  Value=15
  Constant3 : Constant  Value=17
  Gain : Gain  Gain=2.5
  Gain1 : Gain  Gain=5.5
  Gain2 : Gain  Gain=4
  PID Controller : slpidlib/PID Controller  Controller=PID  Form=Parallel  TimeDomain=Continuous-time  UseExternalTs=off  SampleTime=-1  IntegratorMethod=Forward Euler  FilterMethod=Forward Euler  ControllerParametersSource=internal  P=1  I=0.1  UseKiTs=off  D=1  N=100  UseFilter=on  TunerSelectOption=Transfer Function Based (PID Tuner App)  InitialConditionSource=internal  InitialConditionForIntegrator=0  InitialConditionForFilter=0  DifferentiatorICPrevScaledInput=0  ExternalReset=none  TrackingMode=off  Kt=1  LimitOutput=on  SatLimitsSource=internal  UpperSaturationLimit=2.5  LowerSaturationLimit=-2.5  LinearizeAsGain=on  AntiWindupMode=clamping  Kb=1  LimitIntegrator=off  UpperIntegratorSaturationLimit=inf  LowerIntegratorSaturationLimit=-inf  POutMin=[]  POutMax=[]  IOutMin=[]  IOutMax=[]  DOutMin=[]  DOutMax=[]  NOutMin=[]  NOutMax=[]  SumOutMin=[]  SumOutMax=[]  SaturationOutMin=[]  SaturationOutMax=[]  PParamMin=[]  PParamMax=[]  IParamMin=[]  IParamMax=[]  DParamMin=[]  DParamMax=[]  NParamMin=[]  NParamMax=[]  KbParamMin=[]  KbParamMax=[]  KtParamMin=[]  KtParamMax=[]  KbOutMin=[]  KbOutMax=[]  KtOutMin=[]  KtOutMax=[]  IntegratorOutMin=[]  IntegratorOutMax=[]  FilterOutMin=[]  FilterOutMax=[]  SumI1OutMin=[]  SumI1OutMax=[]  SumI2OutMin=[]  SumI2OutMax=[]  SumI3OutMin=[]  SumI3OutMax=[]  SumI4OutMin=[]  SumI4OutMax=[]  SumDOutMin=[]  SumDOutMax=[]  DifferentiatorOutMin=[]  DifferentiatorOutMax=[]  FilterDiffOutCoefMin=[]  FilterDiffOutCoefMax=[]  ReciprocalOutMin=[]  ReciprocalOutMax=[]  SumDenOutMin=[]  SumDenOutMax=[]  SumNumOutMin=[]  SumNumOutMax=[]  DivideOutMin=[]  DivideOutMax=[]  UdiffTsProdOutMin=[]  UdiffTsProdOutMax=[]  NTsProdOutMin=[]  NTsProdOutMax=[]  UintegralTsProdOutMin=[]  UintegralTsProdOutMax=[]  UngainTsProdOutMin=[]  UngainTsProdOutMax=[]  IntegratorContinuousStateAttributes=''  IntegratorStateMustResolveToSignalObject=off  IntegratorRTWStateStorageClass=Auto  FilterContinuousStateAttributes=''  FilterStateMustResolveToSignalObject=off  FilterRTWStateStorageClass=Auto  ParallelPVariant=InternalParameters  IdealPVariant=Disabled  IVariant=InternalParameters  DVariant=InternalParameters  IntegratorVariant=Continuous  SatVariant=Enabled  AWVariant=ContClampingParallel  PCopyVariant=Disabled  TRVariant=Disabled  FdbkBlocksVariant=Forward  IdealPFdbkVariant=Disabled  SatFdbkVariant=Disabled  DerivativeFilterVariant=ContFilter  NVariant=InternalParameters  NCopyVariant=Disabled  FilterICVariant=InternalICsFilter  IntegratorICVariant=InternalICs  ExternalResetVariant=Disabled  TRSumVariant=Passthrough  SumFdbkVariant=Disabled  SumVariant=Sum_PID  TsampFilterVariant=InternalTs  TsampNgainVariant=Passthrough  TsampIntegralVariant=Passthrough  ExternalSaturationOutDataTypeStr=Inherit: Same as second input
  Relational Operator : RelationalOperator  OutDataTypeStr=boolean  RndMeth=Simplest  InputSameDT=off
  Relational Operator1 : RelationalOperator  Operator=<  OutDataTypeStr=boolean  RndMeth=Simplest  InputSameDT=off
  Relational Operator2 : RelationalOperator  OutDataTypeStr=boolean  RndMeth=Simplest  InputSameDT=off
  Relational Operator3 : RelationalOperator  Operator=<  OutDataTypeStr=boolean  RndMeth=Simplest  InputSameDT=off
  Simulink-PS Converter : nesl_utility_internal/Simulink-PS Converter  PhysicalDomain=network_engine_domain  SubClassName=ps_input  LeftPortType=input  RightPortType=output  PseudoPeriodic=off  Frequencies=[]  NoiseDistribution=none  NoiseParameters=[]  Unit=mm  AffineConversion=off  FilteringAndDerivatives=filter  SimscapeFilterOrder=1  InputFilterTimeConstant=0.001  UdotUserProvided=0
  Sum : Sum  Inputs=|+-
  Sum1 : Sum  Inputs=|++
  Sum2 : Sum  Inputs=|+++
  T_environment : Constant  Value=T_env
  T_set : Constant  Value=T_set
  Transfer Fcn (with initial outputs) : simulink_extras/Additional Linear/Transfer Fcn (with initial outputs)  N=[1]  D="[10  1]"  Y0=19  U0=0
  S : PMIOPort  Side=Right
  wires:
  Transfer Fcn (with initial outputs)/1 -> Sum/2
  Sum2/1 -> Sum1/2
  Gain2/1 -> Sum2/3
  Relational Operator3/1 -> AND/2
  Relational Operator2/1 -> AND/1
  AND/1 -> Gain2/1
  Constant3/1 -> Relational Operator3/2
  T_environment/1 -> Relational Operator2/1, Relational Operator3/1, Relational Operator1/1, Relational Operator/1
  Constant2/1 -> Relational Operator2/2
  Gain1/1 -> Sum2/2
  Gain/1 -> Sum2/1
  Constant1/1 -> Relational Operator1/2
  Relational Operator1/1 -> Gain1/1
  Relational Operator/1 -> Gain/1
  Constant/1 -> Relational Operator/2
  Sum1/1 -> Simulink-PS Converter/1
  PID Controller/1 -> Sum1/1
  T/1 -> Transfer Fcn (with initial outputs)/1
  T_set/1 -> Sum/1
  Sum/1 -> PID Controller/1
  connections:
  S/RConn1 -- Simulink-PS Converter/RConn1

== system ElectricalCoolingSystemSSC/Heating-Cooling Unit/Coolant temperature ==
  Absolute Reference (TL) : fl_lib/Thermal Liquid/Elements/Absolute Reference (TL)
  PS-Simulink Converter : nesl_utility_internal/PS-Simulink Converter  PhysicalDomain=network_engine_domain  SubClassName=ps_output  LeftPortType=input  RightPortType=output  PseudoPeriodic=off  Frequencies=[]  VectorFormat=1-D array  Unit=degC  AffineConversion=on
  Pressure & Temperature Sensor (TL) : fl_lib/Thermal Liquid/Sensors/Pressure & Temperature Sensor (TL)
      settings: InternalSimscapePortConfiguration="{\"Bottom\":[],\"Left\":[{\"id\":\"A\",\"label\":\"A\",\"type\":\"foundation.thermal_liquid.thermal_liquid\"}],\"Right\":[{\"id\":\"B\",\"label\":\"B\",\"type\":\"foundation.thermal_liquid.thermal_liquid\"},{\"id\":\"P\",\"label\":\"P\",\"type\":\"output\"},{\"id\":\"T\",\"label\":\"T\",\"type\":\"output\"}],\"Top\":[]}"
  A : PMIOPort  Side=Left
  T : Outport  VectorParamsAs1DForOutWhenUnconnected=off
  wires:
  PS-Simulink Converter/1 -> T/1
  connections:
  Pressure & Temperature Sensor (TL)/LConn1 -- A/RConn1
  Pressure & Temperature Sensor (TL)/RConn3 -- PS-Simulink Converter/LConn1
  Pressure & Temperature Sensor (TL)/RConn1 -- Absolute Reference (TL)/LConn1

== system ElectricalCoolingSystemSSC/Heating-Cooling Unit/Heater ==
  Controlled Temperature Source1 : fl_lib/Thermal/Thermal Sources/Controlled Temperature Source
  Heater Temperature : Subsystem  mask{T_heat=303}
      mask prompts: T_heat "Heater nominal temperature (K)"
  Mass & Energy Flow Rate Sensor (TL) : fl_lib/Thermal Liquid/Sensors/Mass & Energy Flow Rate Sensor (TL)
      settings: InternalSimscapePortConfiguration="{\"Bottom\":[],\"Left\":[{\"id\":\"A\",\"label\":\"A\",\"type\":\"foundation.thermal_liquid.thermal_liquid\"}],\"Right\":[{\"id\":\"B\",\"label\":\"B\",\"type\":\"foundation.thermal_liquid.thermal_liquid\"},{\"id\":\"M\",\"label\":\"M\",\"type\":\"output\"},{\"id\":\"PHI\",\"label\":\"Phi\",\"type\":\"output\"}],\"Top\":[]}"
  Pipe (TL) : fl_lib/Thermal Liquid/Elements/Pipe (TL)  length=pipe.length cm  area=pipe.area cm^2  Dh=pipe.Dh cm  length_add=0 m  roughness=15e-6 m  Re_lam=2000  Re_tur=4000  shape_factor=64  Nu_lam=3.66  dynamic_compressibility=simscape.enum.onoff.on  inertia=simscape.enum.onoff.off  p0=0.101325 MPa  T0=BattTempInit degC  mdot0=0 kg/s
  Power Sensor : Subsystem
  Thermal Reference1 : fl_lib/Thermal/Thermal Elements/Thermal Reference
  B : PMIOPort  Side=Left
  A : PMIOPort  Port=2  Side=Right
  connections:
  Controlled Temperature Source1/RConn1 -- Heater Temperature/RConn1
  Heater Temperature/LConn1 -- Mass & Energy Flow Rate Sensor (TL)/RConn2
  Mass & Energy Flow Rate Sensor (TL)/LConn1 -- A/RConn1
  Thermal Reference1/LConn1 -- Controlled Temperature Source1/RConn2
  Pipe (TL)/RConn1 -- B/RConn1
  Pipe (TL)/LConn1 -- Mass & Energy Flow Rate Sensor (TL)/RConn1
  Power Sensor/LConn1 -- Pipe (TL)/LConn2
  Power Sensor/RConn1 -- Controlled Temperature Source1/LConn1

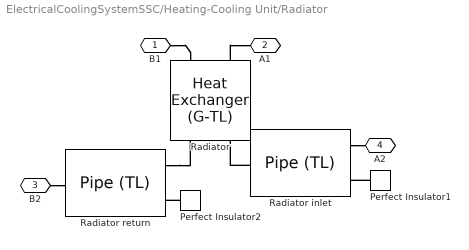
== system ElectricalCoolingSystemSSC/Heating-Cooling Unit/Radiator ==
  Perfect Insulator1 : fl_lib/Thermal/Thermal Elements/Perfect Insulator  T_specify=off  T_priority=None  T=0 K  T_nominal_specify=off  T_nominal_unit=K  T_nominal_value=1
  Perfect Insulator2 : fl_lib/Thermal/Thermal Elements/Perfect Insulator  T_specify=off  T_priority=None  T=0 K  T_nominal_specify=off  T_nominal_unit=K  T_nominal_value=1
  Radiator : SimscapeFluids_lib/Fluid Network Interfaces/Heat Exchangers/Heat Exchanger (G-TL)  hex_type=fluids.interfaces.enum.flow_arrangement_spec.parallel_counter  shell_num=1  cross_type=fluids.interfaces.enum.cross_flow_heat_exchanger_G_TL_spec.mixed_mixed  NTU_TLU=[.5, 1, 2, 3, 4, 5]  CR_TLU=[0, .25, .5, .75, 1]  eff_TLU=[.3, .3, .3, .3, .3; .6, .55, .5, .47, .43; .85, .76, .68, .61, .55; .94, .83, .72, .65, .58; .98, .86, .75, .66, .58; .99, .86, .75, .66, .58]  wall_thermal_dynamics=simscape.enum.onoff.off  thermal_mass_wall=447 J/K  R_wall=1.6e-4 K/W  min_flow_area_1=0.01 m^2  Dh_press_1=0.1 m  gas_volume_1=radiator.volume_air m^3  Re_lam_1=2000  Re_tur_1=4000  pressure_loss_spec_1=fluids.interfaces.enum.pressure_loss_spec.constant  pressure_loss_coeff_1=0.1  length_press_1=1 m  length_add_1=0.1 m  roughness_1=15e-6 m  Re_friction_TLU_1=[400, 1000, 1500, 3000, 4000, 6000, 10000, 20000, 40000, 60000, 100000, 100000000]  friction_factor_TLU_1=[.264, .112, .071, .0417, .0387, .0268, .025, .0232, .0226, .022, .0214, .0214]  shape_factor_1=64  Re_Euler_TLU_1=[50, 500, 1000, 2000]  Euler_TLU_1=[4.4505, .6864, .4791, .3755]  heat_transfer_spec_1=fluids.interfaces.enum.heat_transfer_spec.constant  heat_transfer_area_1=0.4 m^2  heat_coeff_1=100 W/(m^2 * K)  length_heat_1=1 m  Nu_lam_1=3.66  Re_Colburn_TLU_1=[100, 150, 1000]  Colburn_factor_TLU_1=[.019, .013, .002]  Re_Nu_TLU_1=[100, 150, 1000]  Pr_Nu_TLU_1=[1, 10]  Nu_TLU_1=[3.72, 4.21; 3.75, 4.44; 4.21, 7.15]  fouling_factor_1=1e-4 m^2*K/W  mdot_threshold_1=1e-6 kg/s  min_heat_coeff_1=5 W/(m^2 * K)  min_flow_area_2=0.01 m^2  Dh_press_2=0.1 m  liquid_volume_2=radiator.volume_liquid m^3  Re_lam_2=2000  Re_tur_2=4000  pressure_loss_spec_2=fluids.interfaces.enum.pressure_loss_spec.constant  pressure_loss_coeff_2=0.1  length_press_2=1 m  length_add_2=0.1 m  roughness_2=15e-6 m  Re_friction_TLU_2=[400, 1000, 1500, 3000, 4000, 6000, 10000, 20000, 40000, 60000, 100000, 100000000]  friction_factor_TLU_2=[.264, .112, .071, .0417, .0387, .0268, .025, .0232, .0226, .022, .0214, .0214]  shape_factor_2=64  Re_Euler_TLU_2=[50, 500, 1000, 2000]  Euler_TLU_2=[4.4505, .6864, .4791, .3755]  heat_transfer_spec_2=fluids.interfaces.enum.heat_transfer_spec.constant  heat_transfer_area_2=0.4 m^2  heat_coeff_2=100 W/(m^2 * K)  length_heat_2=1 m  Nu_lam_2=3.66  Re_Colburn_TLU_2=[100, 150, 1000]  Colburn_factor_TLU_2=[.019, .013, .002]  Re_Nu_TLU_2=[100, 150, 1000]  Pr_Nu_TLU_2=[1, 10]  Nu_TLU_2=[3.72, 4.21; 3.75, 4.44; 4.21, 7.15]  fouling_factor_2=1e-4 m^2*K/W  min_heat_coeff_2=5 W/(m^2 * K)  T0_1=BattTempInit degC  p0_1=0.105081 %0.101325 MPa  dynamic_compressibility_2=simscape.enum.onoff.on  T0_2=BattTempInit degC  p0_2=0.105081 %0.101325 MPa  mdot1_TLU=radiator.mdot_air kg/s  mdot2_TLU=radiator.mdot_liquid kg/s  SD_TLU=radiator.SD kW/K  Q_check=fluids.interfaces.enum.SD_max_check.none  mdot_dp_TLU_1=radiator.mdot_air kg/s  p_diff_TLU_1=radiator.dp_air MPa  T_ref_in_1=293.15 K  p_ref_in_1=0.101325 MPa  area_1=radiator.area_air m^2  mdot_dp_TLU_2=radiator.mdot_liquid kg/s  p_diff_TLU_2=radiator.dp_liquid MPa  T_ref_in_2=293.15 K  p_ref_in_2=0.101325 MPa  mdot_threshold_2=1e-3 kg/s  area_2=pipe.area cm^2
      settings: InternalSimscapePortConfiguration="{\"Bottom\":[],\"Left\":[{\"id\":\"A1\",\"label\":\"A1\",\"type\":\"foundation.gas.gas\"},{\"id\":\"B1\",\"label\":\"B1\",\"type\":\"foundation.gas.gas\"}],\"Right\":[{\"id\":\"A2\",\"label\":\"A2\",\"type\":\"foundation.thermal_liquid.thermal_liquid\"},{\"id\":\"B2\",\"label\":\"B2\",\"type\":\"foundation.thermal_liquid.thermal_liquid\"}],\"Top\":[]}"
  Radiator inlet : fl_lib/Thermal Liquid/Elements/Pipe (TL)  length=0.25 m  area=pipe.area cm^2  Dh=pipe.Dh cm  length_add=0 m  roughness=15e-6 m  Re_lam=2000  Re_tur=4000  shape_factor=64  Nu_lam=3.66  dynamic_compressibility=simscape.enum.onoff.on  inertia=simscape.enum.onoff.off  p0=0.101325 MPa  T0=BattTempInit degC  mdot0=0 kg/s
  Radiator return : fl_lib/Thermal Liquid/Elements/Pipe (TL)  length=0.25 m  area=pipe.area cm^2  Dh=pipe.Dh cm  length_add=0 m  roughness=15e-6 m  Re_lam=2000  Re_tur=4000  shape_factor=64  Nu_lam=3.66  dynamic_compressibility=simscape.enum.onoff.on  inertia=simscape.enum.onoff.off  p0=0.101325 MPa  T0=BattTempInit degC  mdot0=0 kg/s
  B1 : PMIOPort  Side=Left
  A1 : PMIOPort  Port=2  Side=Right
  B2 : PMIOPort  Port=3  Side=Left
  A2 : PMIOPort  Port=4  Side=Right
  connections:
  B2/RConn1 -- Radiator return/RConn1
  B1/RConn1 -- Radiator/LConn2
  Radiator/LConn1 -- A1/RConn1
  Radiator return/LConn1 -- Radiator/RConn2
  Radiator inlet/LConn1 -- A2/RConn1
  Radiator inlet/RConn1 -- Radiator/RConn1
  Perfect Insulator1/LConn1 -- Radiator inlet/LConn2
  Perfect Insulator2/LConn1 -- Radiator return/LConn2

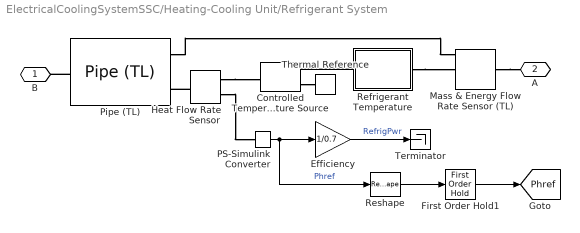
== system ElectricalCoolingSystemSSC/Heating-Cooling Unit/Refrigerant System ==
  Controlled Temperature Source : fl_lib/Thermal/Thermal Sources/Controlled Temperature Source
  Efficiency : Gain  Gain=1/0.7
  First Order Hold1 : FirstOrderHold  ErrorTolerance=inf  AllowContinuousInput=on
  Heat Flow Rate Sensor : fl_lib/Thermal/Thermal Sensors/Heat Flow Rate Sensor
  Mass & Energy Flow Rate Sensor (TL) : fl_lib/Thermal Liquid/Sensors/Mass & Energy Flow Rate Sensor (TL)
      settings: InternalSimscapePortConfiguration="{\"Bottom\":[],\"Left\":[{\"id\":\"A\",\"label\":\"A\",\"type\":\"foundation.thermal_liquid.thermal_liquid\"}],\"Right\":[{\"id\":\"B\",\"label\":\"B\",\"type\":\"foundation.thermal_liquid.thermal_liquid\"},{\"id\":\"M\",\"label\":\"M\",\"type\":\"output\"},{\"id\":\"PHI\",\"label\":\"Phi\",\"type\":\"output\"}],\"Top\":[]}"
  PS-Simulink Converter : nesl_utility_internal/PS-Simulink Converter  PhysicalDomain=network_engine_domain  SubClassName=ps_output  LeftPortType=input  RightPortType=output  PseudoPeriodic=off  Frequencies=[]  VectorFormat=1-D array  Unit=kW  AffineConversion=off
  Pipe (TL) : fl_lib/Thermal Liquid/Elements/Pipe (TL)  length=pipe.length cm  area=pipe.area*10 cm^2  Dh=pipe.Dh cm  length_add=0 m  roughness=15e-6 m  Re_lam=2000  Re_tur=4000  shape_factor=64  Nu_lam=3.66  dynamic_compressibility=simscape.enum.onoff.on  inertia=simscape.enum.onoff.off  p0=0.101325 MPa  T0=BattTempInit degC  mdot0=0 kg/s
  Refrigerant Temperature : Subsystem  mask{T_refrig=274}
      mask prompts: T_refrig "Refrigerant nominal temperature (K)"
  Reshape : Reshape
  Terminator : Terminator
  Thermal Reference : fl_lib/Thermal/Thermal Elements/Thermal Reference
  B : PMIOPort  Side=Left
  A : PMIOPort  Port=2  Side=Right
  tag scope: Phref=global
  wires:
  Efficiency/1 -> Terminator/1  "RefrigPwr"
  PS-Simulink Converter/1 -> Reshape/1, Efficiency/1  "Phref"
  Reshape/1 -> First Order Hold1/1
  First Order Hold1/1 -> [Phref]
  connections:
  Heat Flow Rate Sensor/RConn1 -- PS-Simulink Converter/LConn1
  Heat Flow Rate Sensor/RConn2 -- Controlled Temperature Source/LConn1
  Refrigerant Temperature/RConn1 -- Controlled Temperature Source/RConn1
  Refrigerant Temperature/LConn1 -- Mass & Energy Flow Rate Sensor (TL)/RConn2
  Pipe (TL)/LConn1 -- Mass & Energy Flow Rate Sensor (TL)/RConn1
  Heat Flow Rate Sensor/LConn1 -- Pipe (TL)/LConn2
  Mass & Energy Flow Rate Sensor (TL)/LConn1 -- A/RConn1
  Controlled Temperature Source/RConn2 -- Thermal Reference/LConn1
  Pipe (TL)/RConn1 -- B/RConn1
